simulink model "SimulinkMiniprojekt"  (R2022b)
settings: Solver=VariableStepAuto  StartTime=0.0  StopTime=inf  RelTol=1e-3
model workspace (MAT data in the model file):
  TremoloVar = 1
values from neighbouring files (symbols this model uses):
  D = 20    [MiniprojektMatlabSCRIPT.m]
  sample_frequency = 1/44000    (= 2.27272727273e-05)    [MiniprojektMatlabSCRIPT.m]
libraries: dspsrcs4 x14, dspsigops x2, dspsnks4 x1, dspvision x1
settings Model: SimulationMode=accelerator  Creator=jga-k  LastModifiedBy=jga-k

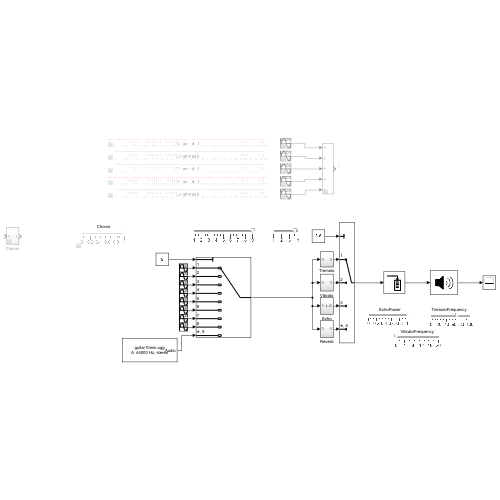
[thumbnail: Simulink's stored preview of the top-level diagram]
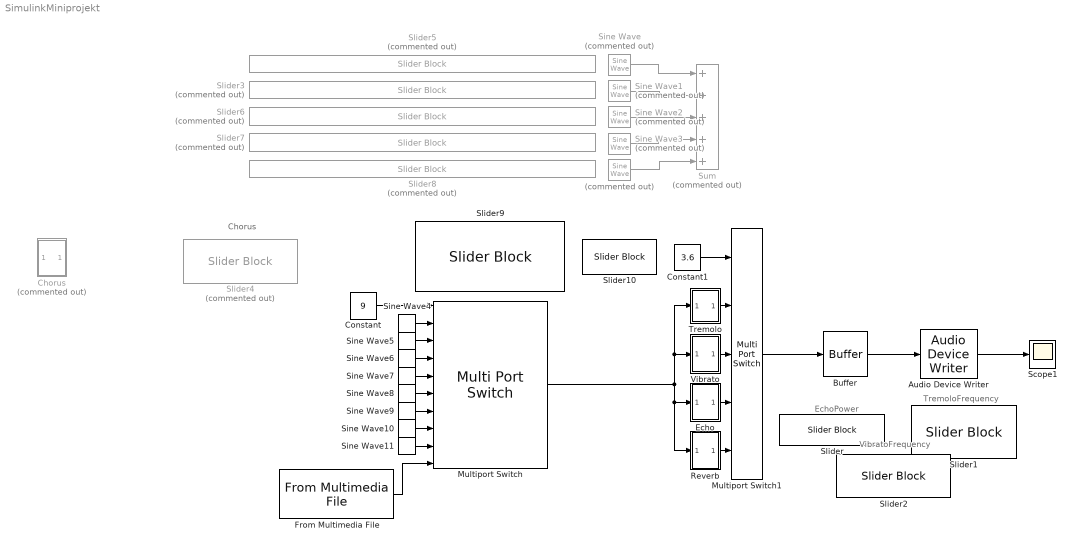
== system SimulinkMiniprojekt ==
  note: Chorus
  note: VibratoFrequency
  note: EchoPower
  note: TremoloFrequency
  " " : dspsrcs4/Sine Wave  Commented=on  Amplitude=1  Frequency=887.3459260445014  Phase=0  SampleMode=Discrete  OutComplex=Real  CompMethod=Trigonometric fcn  TableSize=Speed  SampleTime=1/44100  SamplesPerFrame=1  ResetState=Restart at time zero  OutputFrames=off  dataType=double  wordLen=16  udDataType=sfix(16)  fracBitsMode=Best precision  numFracBits=15  OutDataTypeStr=double  LastOutDataTypeStr=double
  Audio Device Writer : dspsnks4/Audio Device Writer  Driver=DirectSound  Device=Default  InheritSampleRate=off  SampleRate=44000  BitDepth=8-bit integer  BufferSize=4096  NumBuffers=10  DefaultOutputChannelMapping=on  OutputChannelMapping=1:2  OutputNumUnderrunSamples=on  DriverIdx=1  DeviceWarnFlag=''
  Buffer : Buffer  N=500  OutputFrames=off
  Chorus : Subsystem  Commented=on
  Constant : Constant  Value=9
  Constant1 : Constant  Value=3.6
  Echo : Subsystem
  From Multimedia File : dspvision/From Multimedia File  inputFilename=D:\MatLab\toolbox\dsp\samples\guitar10min.ogg  readRange=[1 Inf]  loop=on  numPlays=inf  outputStreams=Audio only  videoDataType=single  audioDataType=double  inheritSampleTime=off  userDefinedSampleTime=sample_frequency  noAudioOutput=off  isIntensityVideo=off  fourcc=RGB  colorVideoFormat=Separate color signals  outputEOF=off  dataOrg=Column-major  audioFrameSize=1  computeAudioFrameSize=off  outSamplingMode=Sample based
      settings: LibrarySourceBlock=audiosources/From Multimedia File
  Multiport Switch : MultiPortSwitch  Inputs=9  SaturateOnIntegerOverflow=off  InputSameDT=off
  Multiport Switch1 : MultiPortSwitch  Inputs=4  SaturateOnIntegerOverflow=off  InputSameDT=off
  Reverb : Subsystem
  Scope1 : Scope
  Sine Wave : dspsrcs4/Sine Wave  Commented=on  Amplitude=1  Frequency=491.635985272931  Phase=0  SampleMode=Discrete  OutComplex=Real  CompMethod=Trigonometric fcn  TableSize=Speed  SampleTime=1/44100  SamplesPerFrame=1  ResetState=Restart at time zero  OutputFrames=off  dataType=double  wordLen=16  udDataType=sfix(16)  fracBitsMode=Best precision  numFracBits=15  OutDataTypeStr=double  LastOutDataTypeStr=double
  Sine Wave1 : dspsrcs4/Sine Wave  Commented=on  Amplitude=1  Frequency=595.3657755722747  Phase=0  SampleMode=Discrete  OutComplex=Real  CompMethod=Trigonometric fcn  TableSize=Speed  SampleTime=1/44100  SamplesPerFrame=1  ResetState=Restart at time zero  OutputFrames=off  dataType=double  wordLen=16  udDataType=sfix(16)  fracBitsMode=Best precision  numFracBits=15  OutDataTypeStr=double  LastOutDataTypeStr=double
  Sine Wave10 : dspsrcs4/Sine Wave  Amplitude=1  Frequency=493.88  Phase=0  SampleMode=Discrete  OutComplex=Real  CompMethod=Trigonometric fcn  TableSize=Speed  SampleTime=sample_frequency  SamplesPerFrame=1  ResetState=Restart at time zero  OutputFrames=off  dataType=double  wordLen=16  udDataType=sfix(16)  fracBitsMode=Best precision  numFracBits=15  OutDataTypeStr=double  LastOutDataTypeStr=double
  Sine Wave11 : dspsrcs4/Sine Wave  Amplitude=1  Frequency=523.25  Phase=0  SampleMode=Discrete  OutComplex=Real  CompMethod=Trigonometric fcn  TableSize=Speed  SampleTime=sample_frequency  SamplesPerFrame=1  ResetState=Restart at time zero  OutputFrames=off  dataType=double  wordLen=16  udDataType=sfix(16)  fracBitsMode=Best precision  numFracBits=15  OutDataTypeStr=double  LastOutDataTypeStr=double
  Sine Wave2 : dspsrcs4/Sine Wave  Commented=on  Amplitude=1  Frequency=700  Phase=0  SampleMode=Discrete  OutComplex=Real  CompMethod=Trigonometric fcn  TableSize=Speed  SampleTime=1/44100  SamplesPerFrame=1  ResetState=Restart at time zero  OutputFrames=off  dataType=double  wordLen=16  udDataType=sfix(16)  fracBitsMode=Best precision  numFracBits=15  OutDataTypeStr=double  LastOutDataTypeStr=double
  Sine Wave3 : dspsrcs4/Sine Wave  Commented=on  Amplitude=1  Frequency=800  Phase=0  SampleMode=Discrete  OutComplex=Real  CompMethod=Trigonometric fcn  TableSize=Speed  SampleTime=1/44100  SamplesPerFrame=1  ResetState=Restart at time zero  OutputFrames=off  dataType=double  wordLen=16  udDataType=sfix(16)  fracBitsMode=Best precision  numFracBits=15  OutDataTypeStr=double  LastOutDataTypeStr=double
  Sine Wave4 : dspsrcs4/Sine Wave  Amplitude=1  Frequency=261.63  Phase=0  SampleMode=Discrete  OutComplex=Real  CompMethod=Trigonometric fcn  TableSize=Speed  SampleTime=sample_frequency  SamplesPerFrame=1  ResetState=Restart at time zero  OutputFrames=off  dataType=double  wordLen=16  udDataType=sfix(16)  fracBitsMode=Best precision  numFracBits=15  OutDataTypeStr=double  LastOutDataTypeStr=double
  Sine Wave5 : dspsrcs4/Sine Wave  Amplitude=1  Frequency=293.66  Phase=0  SampleMode=Discrete  OutComplex=Real  CompMethod=Trigonometric fcn  TableSize=Speed  SampleTime=sample_frequency  SamplesPerFrame=1  ResetState=Restart at time zero  OutputFrames=off  dataType=double  wordLen=16  udDataType=sfix(16)  fracBitsMode=Best precision  numFracBits=15  OutDataTypeStr=double  LastOutDataTypeStr=double
  Sine Wave6 : dspsrcs4/Sine Wave  Amplitude=1  Frequency=329.63  Phase=0  SampleMode=Discrete  OutComplex=Real  CompMethod=Trigonometric fcn  TableSize=Speed  SampleTime=sample_frequency  SamplesPerFrame=1  ResetState=Restart at time zero  OutputFrames=off  dataType=double  wordLen=16  udDataType=sfix(16)  fracBitsMode=Best precision  numFracBits=15  OutDataTypeStr=double  LastOutDataTypeStr=double
  Sine Wave7 : dspsrcs4/Sine Wave  Amplitude=1  Frequency=349.23  Phase=0  SampleMode=Discrete  OutComplex=Real  CompMethod=Trigonometric fcn  TableSize=Speed  SampleTime=sample_frequency  SamplesPerFrame=1  ResetState=Restart at time zero  OutputFrames=off  dataType=double  wordLen=16  udDataType=sfix(16)  fracBitsMode=Best precision  numFracBits=15  OutDataTypeStr=double  LastOutDataTypeStr=double
  Sine Wave8 : dspsrcs4/Sine Wave  Amplitude=1  Frequency=392.00  Phase=0  SampleMode=Discrete  OutComplex=Real  CompMethod=Trigonometric fcn  TableSize=Speed  SampleTime=sample_frequency  SamplesPerFrame=1  ResetState=Restart at time zero  OutputFrames=off  dataType=double  wordLen=16  udDataType=sfix(16)  fracBitsMode=Best precision  numFracBits=15  OutDataTypeStr=double  LastOutDataTypeStr=double
  Sine Wave9 : dspsrcs4/Sine Wave  Amplitude=1  Frequency=440.00  Phase=0  SampleMode=Discrete  OutComplex=Real  CompMethod=Trigonometric fcn  TableSize=Speed  SampleTime=sample_frequency  SamplesPerFrame=1  ResetState=Restart at time zero  OutputFrames=off  dataType=double  wordLen=16  udDataType=sfix(16)  fracBitsMode=Best precision  numFracBits=15  OutDataTypeStr=double  LastOutDataTypeStr=double
  Slider : SliderBlock  LabelPosition=Hide  ScaleMax=1
  Slider1 : SliderBlock  LabelPosition=Hide
  Slider10 : SliderBlock  LabelPosition=Hide  ScaleMin=1  ScaleMax=4
  Slider2 : SliderBlock  LabelPosition=Hide  ScaleMax=20
  Slider{3,5..8} (5 alike) : SliderBlock  Commented=on  LabelPosition=Hide  ScaleMax=1500
  Slider4 : SliderBlock  Commented=on  LabelPosition=Hide  ScaleMax=1
  Slider9 : SliderBlock  LabelPosition=Hide  ScaleMin=1  ScaleMax=9
  Sum : Sum  Commented=on  Inputs=+++++
  Tremolo : Subsystem
  Vibrato : Subsystem
  wires:
  " "/1 -> Sum/5
  Sine Wave3/1 -> Sum/4
  Sine Wave2/1 -> Sum/3
  Sine Wave1/1 -> Sum/2
  Sine Wave/1 -> Sum/1
  Constant/1 -> Multiport Switch/1
  Audio Device Writer/1 -> Scope1/1
  Sine Wave4/1 -> Multiport Switch/2
  Sine Wave5/1 -> Multiport Switch/3
  Sine Wave6/1 -> Multiport Switch/4
  Sine Wave7/1 -> Multiport Switch/5
  Sine Wave8/1 -> Multiport Switch/6
  Sine Wave9/1 -> Multiport Switch/7
  Sine Wave10/1 -> Multiport Switch/8
  Sine Wave11/1 -> Multiport Switch/9
  Tremolo/1(Out1) -> Multiport Switch1/2
  Multiport Switch/1 -> Reverb/1(In1), Echo/1(In1), Vibrato/1(In1), Tremolo/1(In1)
  Constant1/1 -> Multiport Switch1/1
  Multiport Switch1/1 -> Buffer/1
  Buffer/1 -> Audio Device Writer/1
  From Multimedia File/1 -> Multiport Switch/10
  Vibrato/1(Out1) -> Multiport Switch1/3
  Echo/1(Out1) -> Multiport Switch1/4
  Reverb/1(Out1) -> Multiport Switch1/5

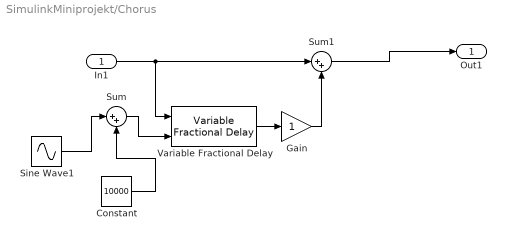
== system SimulinkMiniprojekt/Chorus ==
  In1 : Inport
  Constant : Constant  Value=10000
  Gain : Gain
  Sine Wave1 : Sin  Amplitude=5000  Frequency=100  SampleTime=sample_frequency
  Sum : Sum  Inputs=|++
  Sum1 : Sum  Inputs=|++
  Variable Fractional Delay : dspsigops/Variable Fractional Delay  mode=OBSOLETE  modeActive=Linear  L=4  FarrowL=4  R=10  alpha=1  dmax=100  InputProcessing=Columns as channels (frame based)  ic=0  noDFT=off  fallbackFIR=Clip to the minimum value necessary for centered kernel  fallbackFarrow=Clip to the minimum value necessary for centered kernel  roundingMode=Zero  overflowMode=off
  Out1 : Outport
  wires:
  Sum/1 -> Variable Fractional Delay/2
  Sum1/1 -> Out1/1
  Constant/1 -> Sum/2
  In1/1 -> Sum1/1, Variable Fractional Delay/1
  Sine Wave1/1 -> Sum/1
  Gain/1 -> Sum1/2
  Variable Fractional Delay/1 -> Gain/1

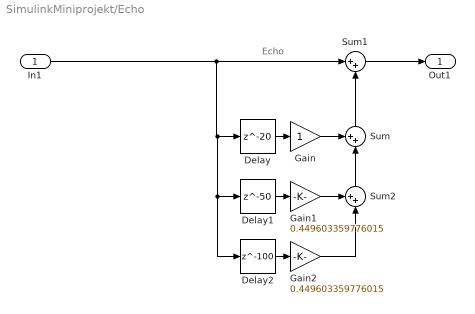
== system SimulinkMiniprojekt/Echo ==
  note: Echo
  In1 : Inport
  Delay : Delay  DelayLength=20  InitialCondition=0
  Delay1 : Delay  DelayLength=50  InitialCondition=0
  Delay2 : Delay  DelayLength=100  InitialCondition=0
  Gain : Gain
  Gain1 : Gain  Gain=0.449603359776015
  Gain2 : Gain  Gain=0.449603359776015
  Sum : Sum  Inputs=++|
  Sum1 : Sum  Inputs=|++
  Sum2 : Sum  Inputs=++|
  Out1 : Outport
  wires:
  Sum1/1 -> Out1/1
  Delay/1 -> Gain/1
  Gain/1 -> Sum/1
  Sum/1 -> Sum1/2
  Gain1/1 -> Sum2/1
  Delay1/1 -> Gain1/1
  Sum2/1 -> Sum/2
  Delay2/1 -> Gain2/1
  In1/1 -> Delay2/1, Delay1/1, Delay/1, Sum1/1
  Gain2/1 -> Sum2/2

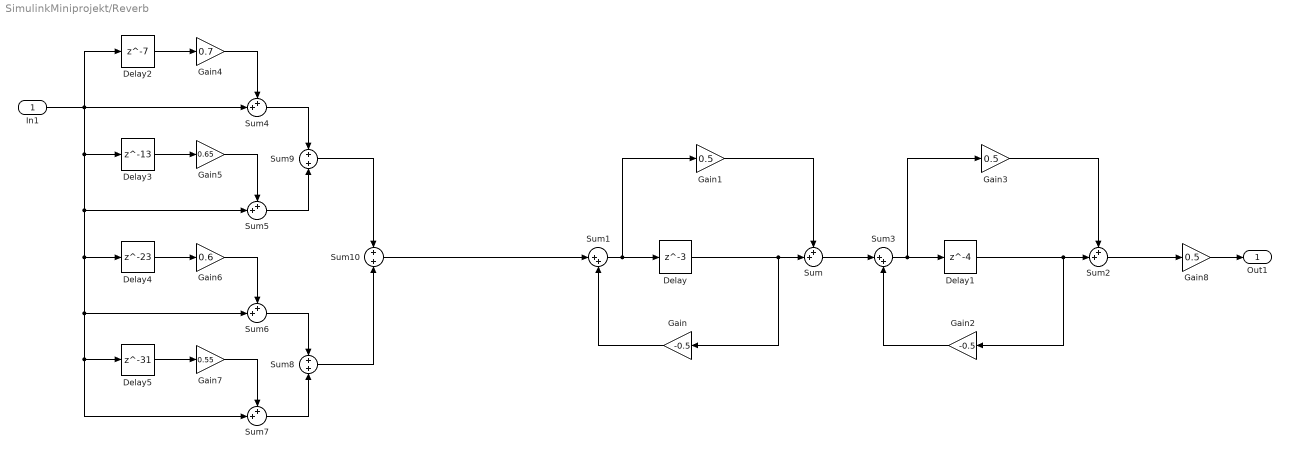
== system SimulinkMiniprojekt/Reverb ==
  In1 : Inport
  Delay : Delay  DelayLength=3
  Delay1 : Delay  DelayLength=4
  Delay2 : Delay  DelayLength=7
  Delay3 : Delay  DelayLength=13
  Delay4 : Delay  DelayLength=23
  Delay5 : Delay  DelayLength=31
  Gain : Gain  Gain=-0.5
  Gain1 : Gain  Gain=0.5
  Gain2 : Gain  Gain=-0.5
  Gain3 : Gain  Gain=0.5
  Gain4 : Gain  Gain=0.7
  Gain5 : Gain  Gain=0.65
  Gain6 : Gain  Gain=0.6
  Gain7 : Gain  Gain=0.55
  Gain8 : Gain  Gain=0.5
  Sum{,2,4..7} (6 alike) : Sum  Inputs=++|
  Sum1 : Sum  Inputs=|++
  Sum10 : Sum
  Sum3 : Sum  Inputs=|++
  Sum8 : Sum
  Sum9 : Sum
  Out1 : Outport
  wires:
  Delay/1 -> Sum/2, Gain/1
  Gain/1 -> Sum1/2
  Sum1/1 -> Gain1/1, Delay/1
  Gain1/1 -> Sum/1
  Sum/1 -> Sum3/1
  Gain3/1 -> Sum2/1
  Sum2/1 -> Gain8/1
  Sum3/1 -> Gain3/1, Delay1/1
  Delay1/1 -> Sum2/2, Gain2/1
  Gain2/1 -> Sum3/2
  Delay2/1 -> Gain4/1
  Gain4/1 -> Sum4/1
  In1/1 -> Sum7/2, Delay5/1, Sum6/2, Delay4/1, Sum5/2, Delay3/1, Sum4/2, Delay2/1
  Delay3/1 -> Gain5/1
  Gain5/1 -> Sum5/1
  Gain6/1 -> Sum6/1
  Delay4/1 -> Gain6/1
  Gain7/1 -> Sum7/1
  Delay5/1 -> Gain7/1
  Sum6/1 -> Sum8/1
  Sum7/1 -> Sum8/2
  Sum4/1 -> Sum9/1
  Sum5/1 -> Sum9/2
  Sum9/1 -> Sum10/1
  Sum8/1 -> Sum10/2
  Sum10/1 -> Sum1/1
  Gain8/1 -> Out1/1

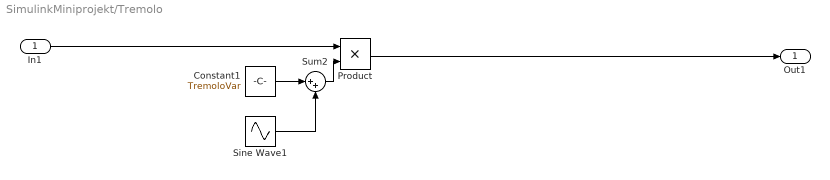
== system SimulinkMiniprojekt/Tremolo ==
  In1 : Inport
  Constant1 : Constant  Value=TremoloVar
  Product : Product
  Sine Wave1 : Sin  Amplitude=TremoloVar  Frequency=67.73215118992067  SampleTime=sample_frequency
  Sum2 : Sum  Inputs=|++
  Out1 : Outport
  wires:
  Sum2/1 -> Product/2
  Constant1/1 -> Sum2/1
  Product/1 -> Out1/1
  In1/1 -> Product/1
  Sine Wave1/1 -> Sum2/2

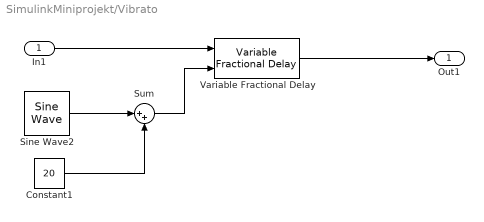
== system SimulinkMiniprojekt/Vibrato ==
  In1 : Inport
  Constant1 : Constant  Value=20
  Sine Wave2 : dspsrcs4/Sine Wave  Amplitude=20  Frequency=0  Phase=0  SampleMode=Discrete  OutComplex=Real  CompMethod=Trigonometric fcn  TableSize=Speed  SampleTime=sample_frequency  SamplesPerFrame=1  ResetState=Restart at time zero  OutputFrames=off  dataType=double  wordLen=16  udDataType=sfix(16)  fracBitsMode=Best precision  numFracBits=15  OutDataTypeStr=double  LastOutDataTypeStr=double
  Sum : Sum  Inputs=|++
  Variable Fractional Delay : dspsigops/Variable Fractional Delay  mode=OBSOLETE  modeActive=Linear  L=4  FarrowL=4  R=10  alpha=1  dmax=100  InputProcessing=Columns as channels (frame based)  ic=0  noDFT=off  fallbackFIR=Clip to the minimum value necessary for centered kernel  fallbackFarrow=Clip to the minimum value necessary for centered kernel  roundingMode=Zero  overflowMode=off
  Out1 : Outport
  wires:
  In1/1 -> Variable Fractional Delay/1
  Sine Wave2/1 -> Sum/1
  Constant1/1 -> Sum/2
  Sum/1 -> Variable Fractional Delay/2
  Variable Fractional Delay/1 -> Out1/1
